simulink model "Subsystem"  (R2020b)
settings: Solver=VariableStepAuto  StartTime=0.0  StopTime=10.0  RelTol=1e-3
settings Model: Creator=Shantam Garg  LastModifiedBy=Shantam Garg
settings DataIOCC: SaveOutput=off  SaveTime=off

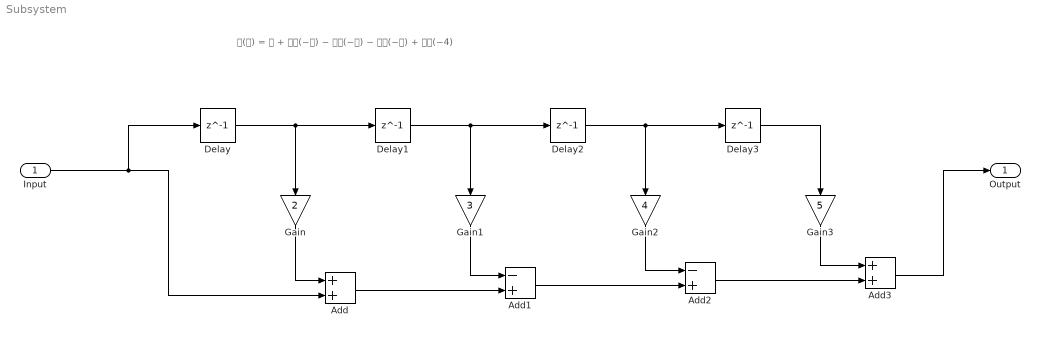
== system Subsystem ==
  note: 𝐇(𝐳) = 𝟏 + 𝟐𝐳(−𝟏) − 𝟑𝐳(−𝟐) − 𝟒𝐳(−𝟑) + 𝟓𝐳(−4)
  Input : Inport  OutDataTypeStr=double  PortDimensions=1  SampleTime=[0,1]
  Add : Sum
  Add1 : Sum  Inputs=-+
  Add2 : Sum  Inputs=-+
  Add3 : Sum
  Delay : Delay  DelayLength=1  InitialCondition=0
  Delay1 : Delay  DelayLength=1
  Delay2 : Delay  DelayLength=1
  Delay3 : Delay  DelayLength=1
  Gain : Gain  Gain=2
  Gain1 : Gain  Gain=3
  Gain2 : Gain  Gain=4
  Gain3 : Gain  Gain=5
  Output : Outport  OutDataTypeStr=double  PortDimensions=1  SampleTime=[0,1]
  wires:
  Input/1 -> Delay/1, Add/2
  Delay1/1 -> Gain1/1, Delay2/1
  Gain1/1 -> Add1/1
  Delay/1 -> Gain/1, Delay1/1
  Delay3/1 -> Gain3/1
  Gain/1 -> Add/1
  Gain2/1 -> Add2/1
  Add/1 -> Add1/2
  Delay2/1 -> Gain2/1, Delay3/1
  Gain3/1 -> Add3/1
  Add1/1 -> Add2/2
  Add2/1 -> Add3/2
  Add3/1 -> Output/1
